simulink model "model3"  (R2019b)
settings: Solver=VariableStepAuto  StartTime=0.0  StopTime=1  RelTol=1e-3
libraries: simulink x2
settings Model: Creator=surtweig  LastModifiedBy=surtweig

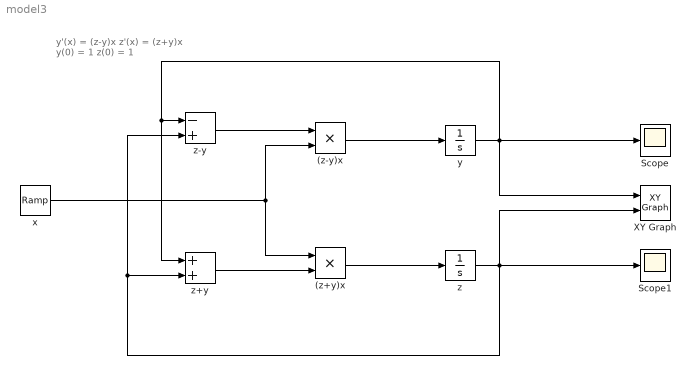
== system model3 ==
  note: y'(x) = (z-y)x
      | z'(x) = (z+y)x
      | y(0) = 1
      | z(0) = 1
  (z+y)x : Product
  (z-y)x : Product
  Scope : Scope
  Scope1 : Scope
  XY Graph : simulink/Sinks/XY Graph  xmin=-3  xmax=3  ymin=-3  ymax=3  st=-1
  x : simulink/Sources/Ramp  slope=1  start=0  InitialOutput=0
  y : Integrator  InitialCondition=1
  z : Integrator  InitialCondition=1
  z+y : Sum
  z-y : Sum  Inputs=-+
  wires:
  z+y/1 -> (z+y)x/2
  z-y/1 -> (z-y)x/1
  x/1 -> (z+y)x/1, (z-y)x/2
  (z-y)x/1 -> y/1
  (z+y)x/1 -> z/1
  z/1 -> XY Graph/2, Scope1/1, z-y/2, z+y/2
  y/1 -> XY Graph/1, Scope/1, z+y/1, z-y/1
